simulink model "QAM_16_Transceiver_Nishat"  (R2018a)
settings: Solver=ode45  StartTime=0.0  StopTime=inf  RelTol=1e-3  EnableMultiTasking=on
values from neighbouring files (symbols this model uses):
  FrameTime = 0.000552    [qpsktxrx16.mat]
  qpsktxrx =     [qpsktxrx16.mat]
undefined symbols (not defined in the file or in its folder): dfilt
libraries: simulink x6, dspsigops x6, dspstat3 x6, dspobslib x6, commdigbbndam3 x5, commblkintrlv2 x5, commutil2 x4, commrflib2 x3, dspsrcs4 x3, commfilt2 x3, commblksprivate x2, dspspect3 x2
(part 2 of 3)

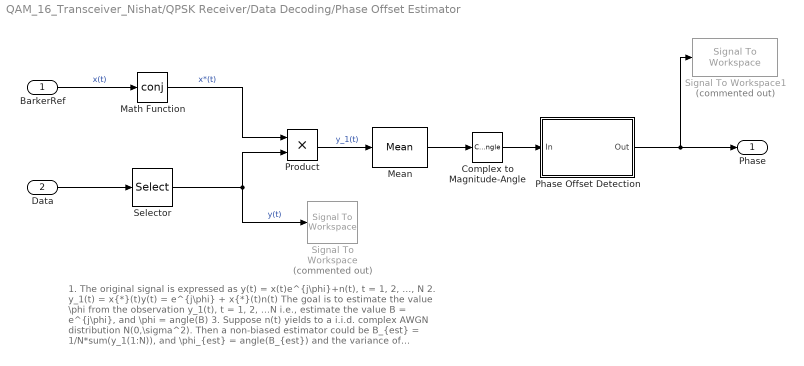
== system QAM_16_Transceiver_Nishat/QPSK Receiver/Data Decoding/Phase Offset Estimator ==
  note: 1. The original signal is expressed as y(t) = x(t)e^{j\phi}+n(t), t = 1, 2, ..., N
      | 2. y_1(t) = x{*}(t)y(t) = e^{j\phi} + x{*}(t)n(t)
      | The goal is to estimate the value \phi from the observation y_1(t), t = 1, 2, ...N
      | i.e., estimate the value B = e^{j\phi}, and \phi = angle(B)
      | 3. Suppose n(t) yields to a i.i.d. complex AWGN distribution N(0,\sigma^2).
      | Then a non-biased estimator could be
      | B_{est} = 1/N*sum(y_1(1:N)), and \phi_{est} = angle(B_{est})
      | and the variance of B_{est} is \sigma^2/N
  BarkerRef : Inport
  Data : Inport  Port=2
  Complex to Magnitude-Angle : ComplexToMagnitudeAngle  Output=Angle
  Math Function : Math  Operator=conj  SaturateOnIntegerOverflow=on
  Mean : dspstat3/Mean  run=off  InputProcessing=Columns as channels (frame based)  reset_popup=None  directionMode=Each column  dimension=1  roiEnable=off  roiType=Rectangles  roiPortion=Entire ROI  roiOutput=Individual statistics for each ROI  roiFlag=off  roundingMode=Floor  overflowMode=off  outputDataTypeStr=Inherit: Same as accumulator  outputMin=[]  outputMax=[]  outputLastDataTypeStr=Inherit: Same as accumulator
  Phase Offset Detection : MATLAB Function  TreatAsAtomicUnit=on
  Product : Product  RndMeth=Zero
  Selector : Selector  IndexOptions=Index vector (dialog)  Indices=[1:26]  OutputSizes=1
  Signal To Workspace : SignalToWorkspace  Commented=on  VariableName=received_Barker
      settings: CopyFcn=dspblkcopystw(gcbh);  Save2DSignal=3-D array (concatenate along third dimension)
  Signal To Workspace1 : SignalToWorkspace  Commented=on  VariableName=Phase_lock_error
      settings: CopyFcn=dspblkcopystw(gcbh);  Save2DSignal=3-D array (concatenate along third dimension)
  Phase : Outport
  wires:
  Data/1 -> Selector/1
  BarkerRef/1 -> Math Function/1  "x(t)"
  Selector/1 -> Product/2, Signal To Workspace/1  "y(t)"
  Math Function/1 -> Product/1  "x*(t)"
  Product/1 -> Mean/1  "y_1(t)"
  Mean/1 -> Complex to Magnitude-Angle/1
  Complex to Magnitude-Angle/1 -> Phase Offset Detection/1(In)
  Phase Offset Detection/1(Out) -> Phase/1, Signal To Workspace1/1

== system QAM_16_Transceiver_Nishat/QPSK Receiver/Fine Frequency Compensation/DDS ==
  note: The digital filter acts as a pure integrator
  In : Inport
  Digital Filter : dspobslib/Digital Filter  TypePopup=IIR (poles & zeros)  IIRFiltStruct=Direct form II transposed  AllPoleFiltStruct=Direct form  FIRFiltStruct=Direct form  CoeffSource=Specify via dialog  NumCoeffs=[0 1]  DenCoeffs=[1 -1]  BiQuadCoeffs=[1 0.3 0.4 1 0.1 0.2]  LatticeCoeffs=[0.2 0.4]  denIgnore=on  FiltPerSampPopup=One filter per frame  IC=0  ICnum=0  ICden=0  roundingMode=Floor  overflowMode=off  ScaleValues=1  scaleValueFracLength=14  stageInFracLength=15  stageOutFracLength=15  FilterSource=Specify via dialog  dfiltObjectName=dfilt.dffir([1 2 1])  InputProcessing=Columns as channels (frame based)
      settings: SourceProductName=DSP System Toolbox  SourceProductBaseCode=DS
  Gain : Gain  Gain=-1*qpsktxrx.PhaseRecoveryGain
  Phase : Outport
  wires:
  Digital Filter/1 -> Gain/1
  In/1 -> Digital Filter/1
  Gain/1 -> Phase/1

== system QAM_16_Transceiver_Nishat/QPSK Receiver/Fine Frequency Compensation/Loop Filter ==
  note: Proportional-plus-Integrator Loop Filter,
      | Infinite DC Response to guarantee convergence
  e : Inport
  Digital Filter : dspobslib/Digital Filter  TypePopup=IIR (poles & zeros)  IIRFiltStruct=Direct form II transposed  AllPoleFiltStruct=Direct form  FIRFiltStruct=Direct form  CoeffSource=Specify via dialog  NumCoeffs=[1 0]  DenCoeffs=[1 -1]  BiQuadCoeffs=[1 0.3 0.4 1 0.1 0.2]  LatticeCoeffs=[0.2 0.4]  denIgnore=on  FiltPerSampPopup=One filter per frame  IC=0  ICnum=0  ICden=0  roundingMode=Floor  overflowMode=off  ScaleValues=1  scaleValueFracLength=14  stageInFracLength=15  stageOutFracLength=15  FilterSource=Specify via dialog  dfiltObjectName=dfilt.dffir([1 2 1])  InputProcessing=Columns as channels (frame based)
      settings: SourceProductName=DSP System Toolbox  SourceProductBaseCode=DS
  K1 : Gain  Gain=K1
  K2 : Gain  Gain=K2
  Sum2 : Sum  SaturateOnIntegerOverflow=on  InputSameDT=on  OutDataTypeStr=Inherit: Same as first input
  v : Outport
  wires:
  K2/1 -> Digital Filter/1
  Digital Filter/1 -> Sum2/2
  Sum2/1 -> v/1
  e/1 -> K2/1, K1/1
  K1/1 -> Sum2/1

== system QAM_16_Transceiver_Nishat/QPSK Receiver/Timing Recovery/Enabled Wire ==
  In : Inport
  Enable : EnablePort
  Out : Outport
  wires:
  In/1 -> Out/1

== system QAM_16_Transceiver_Nishat/QPSK Receiver/Timing Recovery/Modified Buffer ==
  Data : Inport
  Clk : Inport  Port=2
  Frame Conversion : FrameConversion  OutFrame=Sample-based
  Logical Operator : Logic  AllPortsSameDT=off  OutDataTypeStr=boolean
  Modified Buffer : Subsystem
  DataOut : Outport
  DataValid : Outport  Port=2
  wires:
  Data/1 -> Modified Buffer/1(In)
  Modified Buffer/1(DataOut) -> Frame Conversion/1
  Modified Buffer/2(DataValid) -> Logical Operator/1
  Logical Operator/1 -> DataValid/1
  Frame Conversion/1 -> DataOut/1
  Clk/1 -> Modified Buffer/Enable, Logical Operator/2

== system QAM_16_Transceiver_Nishat/QPSK Receiver/Timing Recovery/Timing Recovery PLL ==
  note: Sample-based processing is adopted because
      | 1. Strobe signal is required to generate for EVERY sample for processing and output
      | sampling, delayed strobe signal would affect the accuracy of bit stripping/stuffing
      | 2. The BER performance degrades significantly even with frame size 2 and 4
  note: Baseband implementation of the Symbol Timing Synchronization listed in Chapter 8.4
      | of "Digital Communications- A Discrete-Time Approach" by Michael Rice. See Appendix
      | C.2 of the same book for the details of PLL design.
  note: To determine phase error detector gain K_p, See Equation 8.42 &
      | Figure 8.4.7 of "Digital Communications - A Discrete-Time Approach"
      | by Michael Rice.
  DataIn : Inport
  Integer Delay1 : Delay  DelayLength=1  InputProcessing=Inherited
  Integer Delay2 : Delay  DelayLength=1  InputProcessing=Inherited
  Interpolation Filter : MATLAB Function  TreatAsAtomicUnit=on
  Loop Filter : Subsystem  mask{BnTs=0.01, zeta=1, Kp=qpsktxrx.TimingErrorDetectorGain, K0=qpsktxrx.TimingRecoveryGain, N=qpsktxrx.Upsampling/qpsktxrx.Downsampling}
      mask prompts: BnTs "Loop Bandwidth"; zeta "Loop Damping Factor"; Kp "Phase Detector Gain (Kp)"; K0 "DDS gain (K0)"; N "Number of Samples/symbol (N)"
      mask init:
      | % See C.57 to C.61 in Michael Rice's "Digital Communications 
      | % - A Discrete-Time Approach" for details
      | theta = BnTs/(zeta+0.25/zeta)/N;
      | d = 1 + 2*zeta*theta + theta*theta;
      | K1 = 4*zeta*theta/d;
      | K2 = 4*theta*theta/d;
      | K1 = K1/(Kp*K0);
      | K2 = K2/(Kp*K0);
      mask Display: disp('Loop Filter');
  NCO Control : MATLAB Function
  Normalized Timing Error : Scope
  Timing Error Detector : MATLAB Function  TreatAsAtomicUnit=on
  DataOut : Outport
  ClkOut : Outport  Port=2
  wires:
  DataIn/1 -> Interpolation Filter/1(In)
  NCO Control/2(mu) -> Integer Delay2/1
  Integer Delay1/1 -> ClkOut/1, Timing Error Detector/2(strobe)
  NCO Control/1(Underflow) -> Integer Delay1/1
  Interpolation Filter/1(Out) -> DataOut/1, Timing Error Detector/1(In)
  Loop Filter/1(v) -> NCO Control/1(Delta)
  Timing Error Detector/1(e) -> Loop Filter/1(e)
  Integer Delay2/1 -> Interpolation Filter/2(mu), Normalized Timing Error/1

== system QAM_16_Transceiver_Nishat/Receiver/Coarse Frequency Compensation/Find Frequency Offset ==
  note: This subsystem does the following:
      | 1.  Creates a tone at M*Foffset, where M is the modulation order of the signal
      | 2.  Finds the index of the maximum amplitude across the frequency band
      | 3.  Converts the index to the frequency offset according to
      | Foffset = IndexofMaxAmplitude * FrameSize / (FFTLength * M * FrameSampleTime)
  In : Inport
  Alphabet size : Constant  Value=4  OutDataTypeStr=Inherit: Inherit via back propagation
  Complex Power : commblksprivate/Complex Power
      settings: SourceProductName=Communications System Toolbox  SourceProductBaseCode=CM
  Find Frequency Offset : MATLAB Function  TreatAsAtomicUnit=on
  Periodogram : dspspect3/Periodogram  measurement=Power spectral density  wintype=Hamming  Rs=50  beta=5  winsamp=Symmetric  FFTImplementation=Auto  inheritFFT=off  fftsize=2048  navg=2  inheritTs=on  Ts=1
      settings: SourceProductName=DSP System Toolbox  SourceProductBaseCode=DS
  Probe : Probe  ProbeComplexSignal=off
  Signal To Workspace : SignalToWorkspace  Commented=on  VariableName=width
      settings: CopyFcn=dspblkcopystw(gcbh);  Save2DSignal=3-D array (concatenate along third dimension)
  Freq Offset : Outport
  wires:
  Periodogram/1 -> Find Frequency Offset/3(FFTSig)
  Alphabet size/1 -> Complex Power/2
  In/1 -> Complex Power/1
  Probe/1 -> Find Frequency Offset/1(N)
  Probe/2 -> Find Frequency Offset/2(Tf)
  Find Frequency Offset/1(FreqOffset) -> Signal To Workspace/1, Freq Offset/1
  Complex Power/1 -> Probe/1, Periodogram/1

== system QAM_16_Transceiver_Nishat/Receiver/Data Decoding/Barker Code Symbol Generation  ==
  note: Regenerate a QPSK-modulated unipolar Barker code sequence
      | to be compared with the received data
  Constant Barker Code : Constant  Value=|  VectorParams1D=off  OutDataTypeStr=double
      | [+1 +1 +1 +1 +1 -1 -1 +1 +1 -1 +1 -1 +1
      | ].' > 0
  Matrix Concatenate : Concatenate  Mode=Multidimensional array
  Rectangular QAM Modulator Baseband : commdigbbndam3/Rectangular QAM Modulator Baseband  M=16  InType=Bit  Enc=Gray  Mapping=[0:15]  PowType=Min. distance between symbols  MinDist=2  AvgPow=1  PeakPow=1  Ph=0  outDtype=double  outWordLen=16  outUDDataType=sfix(16)  outFracLenMode=Best precision  outFracLen=15  outDataTypeStr=double  outLastDataTypeStr=double
  Repeat : dspsigops/Repeat  N=4  InputProcessing=Columns as channels (frame based)  RateOptions=Enforce single-rate processing  ic=0  mode=Unused parameter value
      settings: SourceProductName=DSP System Toolbox
  Out : Outport
  wires:
  Constant Barker Code/1 -> Repeat/1
  Repeat/1 -> Rectangular QAM Modulator Baseband/1
  Rectangular QAM Modulator Baseband/1 -> Matrix Concatenate/2, Matrix Concatenate/1
  Matrix Concatenate/1 -> Out/1

== system QAM_16_Transceiver_Nishat/Receiver/Data Decoding/Bit Generation ==
  note: Each data frame contains 26 bits header (For Sync Purpose) and 174 bits data bits,
      | first 105 bits contain "Hello world ###" message. Scrambler is there to improve data
      | transition density and frequency offset estimation.
  Barker Code SS : Subsystem
      mask Display: disp('Unipolar\nBarker Code')
  Frame Conversion : FrameConversion  OutFrame=Sample-based
  Matrix Concatenate : Concatenate  NumInputs=3  Mode=Multidimensional array
  Random Interleaver : commblkintrlv2/Random Interleaver  N=qpsktxrx.DataLength  seed=12345
      settings: SourceProductName=Communications System Toolbox  SourceProductBaseCode=CM
  Repeat : dspsigops/Repeat  N=4  InputProcessing=Columns as channels (frame based)  RateOptions=Enforce single-rate processing  ic=0  mode=Unused parameter value
      settings: SourceProductName=DSP System Toolbox
  Signal From Workspace : dspsrcs4/Signal From Workspace  X=qpsktxrx.sBit2  Ts=-1  nsamps=qpsktxrx.DataLength  OutputAfterFinalValue=Cyclic repetition  ignoreOrWarnInputAndFrameLengths=off  OutputFrames=on
  Out : Outport
  wires:
  Frame Conversion/1 -> Random Interleaver/1
  Repeat/1 -> Matrix Concatenate/2, Matrix Concatenate/1
  Signal From Workspace/1 -> Frame Conversion/1
  Matrix Concatenate/1 -> Out/1
  Barker Code SS/1(Out) -> Repeat/1
  Random Interleaver/1 -> Matrix Concatenate/3

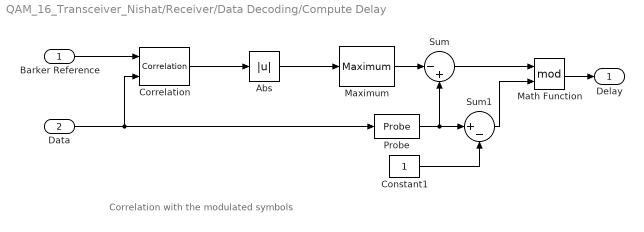
== system QAM_16_Transceiver_Nishat/Receiver/Data Decoding/Compute Delay ==
  note: Correlation with the modulated symbols
  Barker Reference : Inport
  Data : Inport  Port=2
  Abs : Abs
  Constant1 : Constant  VectorParams1D=off  OutDataTypeStr=Inherit: Inherit via back propagation  FramePeriod=2
  Correlation : dspstat3/Correlation  domain=Time  roundingMode=Floor  overflowMode=off  accumDataTypeStr=Inherit: Same as product output  accumLastDataTypeStr=Inherit: Same as product output  outputDataTypeStr=Inherit: Same as accumulator  outputMin=[]  outputMax=[]  outputLastDataTypeStr=Inherit: Same as accumulator
      settings: SourceProductName=DSP System Toolbox  SourceProductBaseCode=DS
  Math Function : Math  Operator=mod  SaturateOnIntegerOverflow=on
  Maximum : dspstat3/Maximum  operation=maximum  fcn=Index  indexBase=One  operateOver=Each column  Dimension=1  InputProcessing=Columns as channels (frame based)  reset=None  roiEnable=off  roiType=Rectangles  roiPortion=Entire ROI  roiOutput=Individual statistics for each ROI  roiFlag=off  roundingMode=Floor  overflowMode=off  accumDataTypeStr=Inherit: Same as product output  accumLastDataTypeStr=Inherit: Same as product output
  Probe : Probe  ProbeSampleTime=off  ProbeComplexSignal=off
  Sum : Sum  Inputs=|-+  SaturateOnIntegerOverflow=on  InputSameDT=on  OutDataTypeStr=Inherit: Same as first input
  Sum1 : Sum  Inputs=|+-  SaturateOnIntegerOverflow=on  InputSameDT=on  OutDataTypeStr=Inherit: Same as first input
  Delay : Outport
  wires:
  Abs/1 -> Maximum/1
  Constant1/1 -> Sum1/2
  Sum1/1 -> Math Function/2
  Math Function/1 -> Delay/1
  Sum/1 -> Math Function/1
  Probe/1 -> Sum1/1, Sum/2
  Correlation/1 -> Abs/1
  Maximum/1 -> Sum/1
  Barker Reference/1 -> Correlation/1
  Data/1 -> Correlation/2, Probe/1

== system QAM_16_Transceiver_Nishat/Receiver/Data Decoding/Descrambling ==
  In : Inport
  Random Deinterleaver : commblkintrlv2/Random Deinterleaver  N=qpsktxrx.DataLength  seed=12345
      settings: SourceProductName=Communications System Toolbox  SourceProductBaseCode=CM
  Selector : Selector  IndexOptions=Index vector (dialog)  Indices=[qpsktxrx.BarkerLength*log2(qpsktxrx.M)+1:qpsktxrx.FrameSize*log2(qpsktxrx.M)]  OutputSizes=1
  Signal To Workspace : SignalToWorkspace  Commented=on  VariableName=after_deinterleaver
      settings: CopyFcn=dspblkcopystw(gcbh);
  Signal To Workspace1 : SignalToWorkspace  Commented=on  VariableName=before_deinterleaver
      settings: CopyFcn=dspblkcopystw(gcbh);
  Signal To Workspace2 : SignalToWorkspace  Commented=on  VariableName=received_complete
      settings: CopyFcn=dspblkcopystw(gcbh);
  Out : Outport
  wires:
  Selector/1 -> Random Deinterleaver/1, Signal To Workspace1/1
  In/1 -> Signal To Workspace2/1, Selector/1
  Random Deinterleaver/1 -> Out/1, Signal To Workspace/1

== system QAM_16_Transceiver_Nishat/Receiver/Data Decoding/Phase Ambiguity Correction & Demodulation ==
  note: Phase Ambiguity Resolution
      | and Demodulation
  Phase : Inport
  Data : Inport  Port=2
  Complex Phase Shift : commutil2/Complex Phase Shift
      settings: SourceProductName=Communications System Toolbox  SourceProductBaseCode=CM
  Corrected Symbols : ConstellationDiagram  Tag=ScatterPlot
  Gain : Gain  Gain=-1  OutDataTypeStr=Inherit: Same as input
  Probe2 : Probe  ProbeSampleTime=off  ProbeComplexSignal=off
  Rectangular QAM Demodulator Baseband : commdigbbndam3/Rectangular QAM Demodulator Baseband  M=16  OutType=Bit  DecType=Hard decision  VarSource=Dialog  Variance=1  Dec=Gray  Mapping=[0:15]  PowType=Min. distance between symbols  MinDist=2  AvgPow=1  PeakPow=1  Ph=0  outDtype1=Inherit via internal rule  outDtype2=Inherit via internal rule  derotateFactorWordLen=16  derotateFactorDataTypeStr=Inherit: Same word length as input  derotateFactorLastDataTypeStr=Inherit: Same word length as input  denormFactorWordLen=16  denormFactorDataTypeStr=Inherit: Same word length as input  denormFactorLastDataTypeStr=Inherit: Same word length as input  prodOutWordLen=32  prodOutOverflowMode=Wrap  prodOutRoundingMode=Floor  prodOutOvFlMode=off  prodOutOvFlModeLastStrValue=off  sumWordLen=32
  Signal To Workspace2 : SignalToWorkspace  Commented=on  VariableName=after_phase_ambiguity
      settings: CopyFcn=dspblkcopystw(gcbh);
  Out : Outport
  wires:
  Phase/1 -> Gain/1
  Complex Phase Shift/1 -> Signal To Workspace2/1, Probe2/1, Corrected Symbols/1, Rectangular QAM Demodulator Baseband/1
  Rectangular QAM Demodulator Baseband/1 -> Out/1
  Gain/1 -> Complex Phase Shift/2
  Data/1 -> Complex Phase Shift/1

== system QAM_16_Transceiver_Nishat/Receiver/Data Decoding/Phase Offset Estimator ==
  note: 1. The original signal is expressed as y(t) = x(t)e^{j\phi}+n(t), t = 1, 2, ..., N
      | 2. y_1(t) = x{*}(t)y(t) = e^{j\phi} + x{*}(t)n(t)
      | The goal is to estimate the value \phi from the observation y_1(t), t = 1, 2, ...N
      | i.e., estimate the value B = e^{j\phi}, and \phi = angle(B)
      | 3. Suppose n(t) yields to a i.i.d. complex AWGN distribution N(0,\sigma^2).
      | Then a non-biased estimator could be
      | B_{est} = 1/N*sum(y_1(1:N)), and \phi_{est} = angle(B_{est})
      | and the variance of B_{est} is \sigma^2/N
  BarkerRef : Inport
  Data : Inport  Port=2
  Complex to Magnitude-Angle : ComplexToMagnitudeAngle  Output=Angle
  Math Function : Math  Operator=conj  SaturateOnIntegerOverflow=on
  Mean : dspstat3/Mean  run=off  InputProcessing=Columns as channels (frame based)  reset_popup=None  directionMode=Each column  dimension=1  roiEnable=off  roiType=Rectangles  roiPortion=Entire ROI  roiOutput=Individual statistics for each ROI  roiFlag=off  roundingMode=Floor  overflowMode=off  outputDataTypeStr=Inherit: Same as accumulator  outputMin=[]  outputMax=[]  outputLastDataTypeStr=Inherit: Same as accumulator
  Phase Offset Detection : MATLAB Function  TreatAsAtomicUnit=on
  Product : Product  RndMeth=Zero
  Selector : Selector  IndexOptions=Index vector (dialog)  Indices=[1:26]  OutputSizes=1
  Signal To Workspace : SignalToWorkspace  Commented=on  VariableName=received_Barker
      settings: CopyFcn=dspblkcopystw(gcbh);  Save2DSignal=3-D array (concatenate along third dimension)
  Signal To Workspace1 : SignalToWorkspace  Commented=on  VariableName=Phase_lock_error
      settings: CopyFcn=dspblkcopystw(gcbh);  Save2DSignal=3-D array (concatenate along third dimension)
  Phase : Outport
  wires:
  Data/1 -> Selector/1
  BarkerRef/1 -> Math Function/1  "x(t)"
  Selector/1 -> Product/2, Signal To Workspace/1  "y(t)"
  Math Function/1 -> Product/1  "x*(t)"
  Product/1 -> Mean/1  "y_1(t)"
  Mean/1 -> Complex to Magnitude-Angle/1
  Complex to Magnitude-Angle/1 -> Phase Offset Detection/1(In)
  Phase Offset Detection/1(Out) -> Phase/1, Signal To Workspace1/1

== system QAM_16_Transceiver_Nishat/Receiver/Fine Frequency Compensation/DDS ==
  note: The digital filter acts as a pure integrator
  In : Inport
  Digital Filter : dspobslib/Digital Filter  TypePopup=IIR (poles & zeros)  IIRFiltStruct=Direct form II transposed  AllPoleFiltStruct=Direct form  FIRFiltStruct=Direct form  CoeffSource=Specify via dialog  NumCoeffs=[0 1]  DenCoeffs=[1 -1]  BiQuadCoeffs=[1 0.3 0.4 1 0.1 0.2]  LatticeCoeffs=[0.2 0.4]  denIgnore=on  FiltPerSampPopup=One filter per frame  IC=0  ICnum=0  ICden=0  roundingMode=Floor  overflowMode=off  ScaleValues=1  scaleValueFracLength=14  stageInFracLength=15  stageOutFracLength=15  FilterSource=Specify via dialog  dfiltObjectName=dfilt.dffir([1 2 1])  InputProcessing=Columns as channels (frame based)
      settings: SourceProductName=DSP System Toolbox  SourceProductBaseCode=DS
  Gain : Gain  Gain=-1*qpsktxrx.PhaseRecoveryGain
  Phase : Outport
  wires:
  Digital Filter/1 -> Gain/1
  In/1 -> Digital Filter/1
  Gain/1 -> Phase/1

== system QAM_16_Transceiver_Nishat/Receiver/Fine Frequency Compensation/Loop Filter ==
  note: Proportional-plus-Integrator Loop Filter,
      | Infinite DC Response to guarantee convergence
  e : Inport
  Digital Filter : dspobslib/Digital Filter  TypePopup=IIR (poles & zeros)  IIRFiltStruct=Direct form II transposed  AllPoleFiltStruct=Direct form  FIRFiltStruct=Direct form  CoeffSource=Specify via dialog  NumCoeffs=[1 0]  DenCoeffs=[1 -1]  BiQuadCoeffs=[1 0.3 0.4 1 0.1 0.2]  LatticeCoeffs=[0.2 0.4]  denIgnore=on  FiltPerSampPopup=One filter per frame  IC=0  ICnum=0  ICden=0  roundingMode=Floor  overflowMode=off  ScaleValues=1  scaleValueFracLength=14  stageInFracLength=15  stageOutFracLength=15  FilterSource=Specify via dialog  dfiltObjectName=dfilt.dffir([1 2 1])  InputProcessing=Columns as channels (frame based)
      settings: SourceProductName=DSP System Toolbox  SourceProductBaseCode=DS
  K1 : Gain  Gain=K1
  K2 : Gain  Gain=K2
  Sum2 : Sum  SaturateOnIntegerOverflow=on  InputSameDT=on  OutDataTypeStr=Inherit: Same as first input
  v : Outport
  wires:
  K2/1 -> Digital Filter/1
  Digital Filter/1 -> Sum2/2
  Sum2/1 -> v/1
  e/1 -> K2/1, K1/1
  K1/1 -> Sum2/1

== system QAM_16_Transceiver_Nishat/Receiver/Timing Recovery/Enabled Wire ==
  In : Inport
  Enable : EnablePort
  Out : Outport
  wires:
  In/1 -> Out/1

== system QAM_16_Transceiver_Nishat/Receiver/Timing Recovery/Modified Buffer ==
  Data : Inport
  Clk : Inport  Port=2
  Frame Conversion : FrameConversion  OutFrame=Sample-based
  Logical Operator : Logic  AllPortsSameDT=off  OutDataTypeStr=boolean
  Modified Buffer : Subsystem
  DataOut : Outport
  DataValid : Outport  Port=2
  wires:
  Data/1 -> Modified Buffer/1(In)
  Modified Buffer/1(DataOut) -> Frame Conversion/1
  Modified Buffer/2(DataValid) -> Logical Operator/1
  Logical Operator/1 -> DataValid/1
  Frame Conversion/1 -> DataOut/1
  Clk/1 -> Modified Buffer/Enable, Logical Operator/2

== system QAM_16_Transceiver_Nishat/Receiver/Timing Recovery/Timing Recovery PLL ==
  note: Sample-based processing is adopted because
      | 1. Strobe signal is required to generate for EVERY sample for processing and output
      | sampling, delayed strobe signal would affect the accuracy of bit stripping/stuffing
      | 2. The BER performance degrades significantly even with frame size 2 and 4
  note: Baseband implementation of the Symbol Timing Synchronization listed in Chapter 8.4
      | of "Digital Communications- A Discrete-Time Approach" by Michael Rice. See Appendix
      | C.2 of the same book for the details of PLL design.
  note: To determine phase error detector gain K_p, See Equation 8.42 &
      | Figure 8.4.7 of "Digital Communications - A Discrete-Time Approach"
      | by Michael Rice.
  DataIn : Inport
  Integer Delay1 : Delay  DelayLength=1  InputProcessing=Inherited
  Integer Delay2 : Delay  DelayLength=1  InputProcessing=Inherited
  Interpolation Filter : MATLAB Function  TreatAsAtomicUnit=on
  Loop Filter : Subsystem  mask{BnTs=0.01, zeta=1, Kp=qpsktxrx.TimingErrorDetectorGain, K0=qpsktxrx.TimingRecoveryGain, N=qpsktxrx.Upsampling/qpsktxrx.Downsampling}
      mask prompts: BnTs "Loop Bandwidth"; zeta "Loop Damping Factor"; Kp "Phase Detector Gain (Kp)"; K0 "DDS gain (K0)"; N "Number of Samples/symbol (N)"
      mask init: same as QAM_16_Transceiver_Nishat/QPSK Receiver/Timing Recovery/Timing Recovery PLL/Loop Filter
      mask Display: disp('Loop Filter');
  NCO Control : MATLAB Function
  Normalized Timing Error : Scope
  Timing Error Detector : MATLAB Function  TreatAsAtomicUnit=on
  DataOut : Outport
  ClkOut : Outport  Port=2
  wires:
  DataIn/1 -> Interpolation Filter/1(In)
  NCO Control/2(mu) -> Integer Delay2/1
  Integer Delay1/1 -> ClkOut/1, Timing Error Detector/2(strobe)
  NCO Control/1(Underflow) -> Integer Delay1/1
  Interpolation Filter/1(Out) -> DataOut/1, Timing Error Detector/1(In)
  Loop Filter/1(v) -> NCO Control/1(Delta)
  Timing Error Detector/1(e) -> Loop Filter/1(e)
  Integer Delay2/1 -> Interpolation Filter/2(mu), Normalized Timing Error/1

== system QAM_16_Transceiver_Nishat/Transmitter/Bit Generation/Barker Code SS ==
  Constant Barker Code : Constant  Value=|  VectorParams1D=off  OutDataTypeStr=double
      | [+1 +1 +1 +1 +1 -1 -1 +1 +1 -1 +1 -1 +1
      | ].' > 0  % Bipolar to Unipolar Conversion
  Out : Outport
  wires:
  Constant Barker Code/1 -> Out/1

== system QAM_16_Transceiver_Nishat/QPSK Receiver/Data Decoding/Bit Generation/Barker Code SS ==
  Constant Barker Code : Constant  Value=|  VectorParams1D=off  OutDataTypeStr=double
      | [+1 +1 +1 +1 +1 -1 -1 +1 +1 -1 +1 -1 +1
      | ].' > 0  % Bipolar to Unipolar Conversion
  Out : Outport
  wires:
  Constant Barker Code/1 -> Out/1

== system QAM_16_Transceiver_Nishat/QPSK Receiver/Timing Recovery/Modified Buffer/Modified Buffer ==
  In : Inport
  Enable : EnablePort
  Compare To Constant : simulink/Logic and Bit Operations/Compare To Constant  relop===  const=(bufSize-1)  OutDataTypeStr=boolean  ZeroCross=off
  Counter Limited : simulink/Sources/Counter Limited  uplimit=(bufSize-1)  tsamp=-1
  Delay Line : dspbuff3/Delay Line  siz=bufSize  ic=0  directfeed=on  enable_output=on  hold_output=off  OutputFrames=on
      settings: SourceProductName=DSP System Toolbox  SourceProductBaseCode=DS
  DataOut : Outport
  DataValid : Outport  Port=2
  wires:
  Compare To Constant/1 -> Delay Line/2, DataValid/1
  Delay Line/1 -> DataOut/1
  In/1 -> Delay Line/1
  Counter Limited/1 -> Compare To Constant/1

== system QAM_16_Transceiver_Nishat/QPSK Receiver/Timing Recovery/Timing Recovery PLL/Loop Filter ==
  note: Proportional-Plus-Integrator Loop Filter,
      | Infinite DC Response to guarantee convergence
  e : Inport
  Digital Filter : dspobslib/Digital Filter  TypePopup=IIR (poles & zeros)  IIRFiltStruct=Direct form II transposed  AllPoleFiltStruct=Direct form  FIRFiltStruct=Direct form  CoeffSource=Specify via dialog  NumCoeffs=[1 0]  DenCoeffs=[1 -1]  BiQuadCoeffs=[1 0.3 0.4 1 0.1 0.2]  LatticeCoeffs=[0.2 0.4]  denIgnore=on  FiltPerSampPopup=One filter per frame  IC=0  ICnum=0  ICden=0  roundingMode=Floor  overflowMode=off  ScaleValues=1  scaleValueFracLength=14  stageInFracLength=15  stageOutFracLength=15  FilterSource=Specify via dialog  dfiltObjectName=dfilt.dffir([1 2 1])  InputProcessing=Columns as channels (frame based)
      settings: SourceProductName=DSP System Toolbox  SourceProductBaseCode=DS
  K1 : Gain  Gain=K1
  K2 : Gain  Gain=K2
  Sum2 : Sum  SaturateOnIntegerOverflow=on  InputSameDT=on  OutDataTypeStr=Inherit: Same as first input
  v : Outport
  wires:
  K2/1 -> Digital Filter/1
  Digital Filter/1 -> Sum2/2
  Sum2/1 -> v/1
  e/1 -> K2/1, K1/1
  K1/1 -> Sum2/1

== system QAM_16_Transceiver_Nishat/Receiver/Data Decoding/Bit Generation/Barker Code SS ==
  Constant Barker Code : Constant  Value=|  VectorParams1D=off  OutDataTypeStr=double
      | [+1 +1 +1 +1 +1 -1 -1 +1 +1 -1 +1 -1 +1
      | ].' > 0  % Bipolar to Unipolar Conversion
  Out : Outport
  wires:
  Constant Barker Code/1 -> Out/1

== system QAM_16_Transceiver_Nishat/Receiver/Timing Recovery/Modified Buffer/Modified Buffer ==
  In : Inport
  Enable : EnablePort
  Compare To Constant : simulink/Logic and Bit Operations/Compare To Constant  relop===  const=(bufSize-1)  OutDataTypeStr=boolean  ZeroCross=off
  Counter Limited : simulink/Sources/Counter Limited  uplimit=(bufSize-1)  tsamp=-1
  Delay Line : dspbuff3/Delay Line  siz=bufSize  ic=0  directfeed=on  enable_output=on  hold_output=off  OutputFrames=on
      settings: SourceProductName=DSP System Toolbox  SourceProductBaseCode=DS
  DataOut : Outport
  DataValid : Outport  Port=2
  wires:
  Compare To Constant/1 -> Delay Line/2, DataValid/1
  Delay Line/1 -> DataOut/1
  In/1 -> Delay Line/1
  Counter Limited/1 -> Compare To Constant/1

== system QAM_16_Transceiver_Nishat/Receiver/Timing Recovery/Timing Recovery PLL/Loop Filter ==
  note: Proportional-Plus-Integrator Loop Filter,
      | Infinite DC Response to guarantee convergence
  e : Inport
  Digital Filter : dspobslib/Digital Filter  TypePopup=IIR (poles & zeros)  IIRFiltStruct=Direct form II transposed  AllPoleFiltStruct=Direct form  FIRFiltStruct=Direct form  CoeffSource=Specify via dialog  NumCoeffs=[1 0]  DenCoeffs=[1 -1]  BiQuadCoeffs=[1 0.3 0.4 1 0.1 0.2]  LatticeCoeffs=[0.2 0.4]  denIgnore=on  FiltPerSampPopup=One filter per frame  IC=0  ICnum=0  ICden=0  roundingMode=Floor  overflowMode=off  ScaleValues=1  scaleValueFracLength=14  stageInFracLength=15  stageOutFracLength=15  FilterSource=Specify via dialog  dfiltObjectName=dfilt.dffir([1 2 1])  InputProcessing=Columns as channels (frame based)
      settings: SourceProductName=DSP System Toolbox  SourceProductBaseCode=DS
  K1 : Gain  Gain=K1
  K2 : Gain  Gain=K2
  Sum2 : Sum  SaturateOnIntegerOverflow=on  InputSameDT=on  OutDataTypeStr=Inherit: Same as first input
  v : Outport
  wires:
  K2/1 -> Digital Filter/1
  Digital Filter/1 -> Sum2/2
  Sum2/1 -> v/1
  e/1 -> K2/1, K1/1
  K1/1 -> Sum2/1

== matlab function QAM_16_Transceiver_Nishat/QPSK Receiver/Auto correlation ==
  data: frame input; frame_length input; output output; auto_corr_length input; Status_value output; Status_position output; MaximumValue output; SecondMaximumValue output; Index output; MaximumIndex output; correction_factor output
 function [output , Status_value , Status_position , MaximumValue , SecondMaximumValue , Index , MaximumIndex , correction_factor]  = auto_corr(frame , frame_length , auto_corr_length)

% This block is data aided preamble based AGC. This can work with any M-QAM
% constellation.

output = complex(zeros(552,1));
frame = frame.';

num_auto_corr = frame_length - 2*auto_corr_length + 1;
assert(num_auto_corr < 2048);
auto_corr_array = complex(zeros(1,num_auto_corr));
auto_corr_array_mag = zeros(1,num_auto_corr);

temp = complex(0);

for i = 1:num_auto_corr
    
    if (i==1)
    
        auto_corr_array(i) = temp + frame(i:auto_corr_length)*((frame(auto_corr_length + i : 2*auto_corr_length)))';    % " ' " used to avoid using sum --> multiplicatin of row and column array
        auto_corr_array_mag(i) = abs(auto_corr_array(i));
        
        temp = auto_corr_array(i) - ( frame(i) * conj(frame(auto_corr_length+i)) );
    
    elseif (i > 1 )
        
        auto_corr_array(i) = temp + (frame(i-1 + auto_corr_length) * conj(frame(i-1 + auto_corr_length*2)) );    % i-1 bcoz when i = 2 then 14 sample should be * with 27 sample not 15 with 28 
        auto_corr_array_mag(i) = abs(auto_corr_array(i));
        
        temp = auto_corr_array(i) - (frame(i) * conj(frame(auto_corr_length + i)) );
    
    else
        disp('NARGIN ERROR ;)');
    end

end

%% confirmation and estimation process
Status_value = 1;
Status_position = 1;
temp_auto_mag = auto_corr_array_mag;

[MaximumValue, MaximumIndex] = max(temp_auto_mag);
MinThresholdIndex = MaximumIndex;
MaxThresholdIndex = MaximumIndex;

Threshold = 0.8*MaximumValue;

LengthData = num_auto_corr;

temp_auto_mag(MaximumIndex) = -100;

for Index = 1:LengthData
    
    if MinThresholdIndex ~= MaximumIndex && MaxThresholdIndex ~= MaximumIndex
        break;
    end
    
    if MaximumIndex-Index >= 1 && MinThresholdIndex == MaximumIndex && temp_auto_mag(MaximumIndex-Index) < Threshold
        MinThresholdIndex = MaximumIndex-Index+1;
    else
        if MinThresholdIndex == MaximumIndex  && MaximumIndex-Index >= 1
        temp_auto_mag(MaximumIndex-Index) = -100;
        end
    end
    
    if MaximumIndex+Index <= LengthData && MaxThresholdIndex == MaximumIndex && temp_auto_mag(MaximumIndex+Index) < Threshold
        MaxThresholdIndex = MaximumIndex+Index-1;
    else
        if MaxThresholdIndex == MaximumIndex && MaximumIndex+Index <= LengthData
        temp_auto_mag(MaximumIndex+Index) = -100;
        end
    end
    
end



[SecondMaximumValue, Index] = max(temp_auto_mag);

if temp_auto_mag(Index) < 0.85*MaximumValue || temp_auto_mag(Index) > 1.15*MaximumValue
    fprintf('ERROR: Large Difference in Preamble Cross Corelation Values\n');
    Status_value = 0;
end

if abs(Index-MaximumIndex) < (frame_length/2 - 16) || abs(Index-MaximumIndex) > (frame_length/2 + 16)
    fprintf('ERROR: Preamlbe Positions Mismatach\n');
    Status_position = 0;
end
% the value of 212 is chosen because it is the autocorrelation for reference constellation
correction_factor = sqrt(complex(212/(SecondMaximumValue + MaximumValue))); %sqrt because a factor alpha in mag transslated to alpha^2 in auto
correction_factor = real(correction_factor); 

output = (frame.')*correction_factor;%/correction_factor;

return;

end

== matlab function QAM_16_Transceiver_Nishat/Channel model/MATLAB Function ==
  data: u input; y output
function y = ChannelMag(u)
% Rangom channel magnitude for each iteration
scale = 1+.1*rand;

y = u*scale;

== matlab function QAM_16_Transceiver_Nishat/Receiver/Auto correlation ==
  data: frame input; frame_length input; output output; auto_corr_length input; Status_value output; Status_position output; MaximumValue output; SecondMaximumValue output; Index output; MaximumIndex output; correction_factor output
 function [output , Status_value , Status_position , MaximumValue , SecondMaximumValue , Index , MaximumIndex , correction_factor]  = auto_corr(frame , frame_length , auto_corr_length)

% This block is data aided preamble based AGC. This can work with any M-QAM
% constellation.

output = complex(zeros(552,1));
frame = frame.';

num_auto_corr = frame_length - 2*auto_corr_length + 1;
assert(num_auto_corr < 2048);
auto_corr_array = complex(zeros(1,num_auto_corr));
auto_corr_array_mag = zeros(1,num_auto_corr);

temp = complex(0);

for i = 1:num_auto_corr
    
    if (i==1)
    
        auto_corr_array(i) = temp + frame(i:auto_corr_length)*((frame(auto_corr_length + i : 2*auto_corr_length)))';    % " ' " used to avoid using sum --> multiplicatin of row and column array
        auto_corr_array_mag(i) = abs(auto_corr_array(i));
        
        temp = auto_corr_array(i) - ( frame(i) * conj(frame(auto_corr_length+i)) );
    
    elseif (i > 1 )
        
        auto_corr_array(i) = temp + (frame(i-1 + auto_corr_length) * conj(frame(i-1 + auto_corr_length*2)) );    % i-1 bcoz when i = 2 then 14 sample should be * with 27 sample not 15 with 28 
        auto_corr_array_mag(i) = abs(auto_corr_array(i));
        
        temp = auto_corr_array(i) - (frame(i) * conj(frame(auto_corr_length + i)) );
    
    else
        disp('NARGIN ERROR ;)');
    end

end

%% confirmation and estimation process
Status_value = 1;
Status_position = 1;
temp_auto_mag = auto_corr_array_mag;

[MaximumValue, MaximumIndex] = max(temp_auto_mag);
MinThresholdIndex = MaximumIndex;
MaxThresholdIndex = MaximumIndex;

Threshold = 0.8*MaximumValue;

LengthData = num_auto_corr;

temp_auto_mag(MaximumIndex) = -100;

for Index = 1:LengthData
    
    if MinThresholdIndex ~= MaximumIndex && MaxThresholdIndex ~= MaximumIndex
        break;
    end
    
    if MaximumIndex-Index >= 1 && MinThresholdIndex == MaximumIndex && temp_auto_mag(MaximumIndex-Index) < Threshold
        MinThresholdIndex = MaximumIndex-Index+1;
    else
        if MinThresholdIndex == MaximumIndex  && MaximumIndex-Index >= 1
        temp_auto_mag(MaximumIndex-Index) = -100;
        end
    end
    
    if MaximumIndex+Index <= LengthData && MaxThresholdIndex == MaximumIndex && temp_auto_mag(MaximumIndex+Index) < Threshold
        MaxThresholdIndex = MaximumIndex+Index-1;
    else
        if MaxThresholdIndex == MaximumIndex && MaximumIndex+Index <= LengthData
        temp_auto_mag(MaximumIndex+Index) = -100;
        end
    end
    
end



[SecondMaximumValue, Index] = max(temp_auto_mag);

if temp_auto_mag(Index) < 0.85*MaximumValue || temp_auto_mag(Index) > 1.15*MaximumValue
    fprintf('ERROR: Large Difference in Preamble Cross Corelation Values\n');
    Status_value = 0;
end

if abs(Index-MaximumIndex) < (frame_length/2 - 16) || abs(Index-MaximumIndex) > (frame_length/2 + 16)
    fprintf('ERROR: Preamlbe Positions Mismatach\n');
    Status_position = 0;
end
% the value of 212 is chosen because it is the autocorrelation for reference constellation
correction_factor = sqrt(complex(212/(SecondMaximumValue + MaximumValue))); %sqrt because a factor alpha in mag transslated to alpha^2 in auto
correction_factor = real(correction_factor); 

output = (frame.')*correction_factor;%/correction_factor;

return;

end

== matlab function QAM_16_Transceiver_Nishat/Receiver/Timing Recovery/Calculate Number of Valid Samples ==
  data: Clk input; numValid output
function numValid = numValidCalc(Clk)
% Calculate the number of valid outputs in the current received frame. The
% typical value is 100 valid outputs in a 200-element frame. However, in
% bit stuffing case we have 101 valid outputs, and in bit stripping case we 
% have 99 valid outputs.
%
% Input:
%   Clk - Strobe signal
% Output:
%   NumValid - Number of valid outputs in the current received frame 
%#codegen
numValid = sum(Clk~=0);

== matlab function QAM_16_Transceiver_Nishat/QPSK Receiver/Coarse Frequency Compensation/Find Frequency Offset/Find Frequency Offset ==
  data: N input; FreqOffset output; Tf input; FFTSig input; qpsktxrx parameter
function FreqOffset  = findfreqoffset(N, Tf, FFTSig, qpsktxrx)
% Find frequency offset
% Input:
%   N - Frame size
%   Tf - Two-element vector:  [Frame time, Offset time]
%   FFTSig - Result of FFT
%   M - Modulation alphabet size
% Output:
%   FreqOffset - Estimated frequency offset
%#codegen

M = qpsktxrx.M; 
FFTSize = length(FFTSig);
FFTSig = fftshift(FFTSig);
[~, maxIdx] = max(FFTSig); % Find index of max magnitude
OffsetIdx = maxIdx-1-FFTSize/2; % Convert to index symmetric with 0
Ts = Tf(1)/N; % Sample time
delta_f = 1/Ts/FFTSize; % Frequency resolution of FFT 
FreqOffset = OffsetIdx*delta_f/4;% Map offset index back to frequency

== matlab function QAM_16_Transceiver_Nishat/QPSK Receiver/Data Decoding/Align Data ==
  data: Delay input; RxData input; Data output
function Data  = aligndata(Delay, RxData)
% Extract data from the buffered RxData, using the delay to find the frame 


Data = RxData(Delay+1:Delay+length(RxData)/2);

== matlab function QAM_16_Transceiver_Nishat/Receiver/Coarse Frequency Compensation/Find Frequency Offset/Find Frequency Offset ==
  data: N input; FreqOffset output; Tf input; FFTSig input; qpsktxrx parameter
function FreqOffset  = findfreqoffset(N, Tf, FFTSig, qpsktxrx)
% Find frequency offset
% Input:
%   N - Frame size
%   Tf - Two-element vector:  [Frame time, Offset time]
%   FFTSig - Result of FFT
%   M - Modulation alphabet size
% Output:
%   FreqOffset - Estimated frequency offset
%#codegen

M = qpsktxrx.M; 
FFTSize = length(FFTSig);
FFTSig = fftshift(FFTSig);
[~, maxIdx] = max(FFTSig); % Find index of max magnitude
OffsetIdx = maxIdx-1-FFTSize/2; % Convert to index symmetric with 0
Ts = Tf(1)/N; % Sample time
delta_f = 1/Ts/FFTSize; % Frequency resolution of FFT 
FreqOffset = OffsetIdx*delta_f/4;% Map offset index back to frequency

== matlab function QAM_16_Transceiver_Nishat/Receiver/Data Decoding/Phase Offset Estimator/Phase Offset Detection ==
  data: In input; Out output
function Out = phasedecision(In)
% Map the estimated phase to one of -pi, -pi/2, 0, pi/2,  
%#codegen
Out = round(In.*2./pi)./2.*pi;
% The above processing is equivalent to the following processing using
% if/else statements
%
% if In<pi/4 && In>-pi/4
%     Out = 0;
% elseif In>=pi/4 && In<pi*3/4
%     Out = pi/2;
% elseif In>=pi*3/4 || In<=-pi*3/4
%     Out = -pi;
% else
%     Out = -pi/2;
% end

== matlab function QAM_16_Transceiver_Nishat/Receiver/Fine Frequency Compensation/PED ==
  data: In input; e output
function e = PED(In)
% Implementation of Maximum Likelihood Phase Error Detector listed in
% Chapter 7.2.2 of "Digital Communications - A Discrete-Time Approach" by
% Michael Rice. This employs a decision directed method.
%
% Input:
%   In - Input samples, oversampled by two
% Output:
%   e - Phase error, de
%#codegen
M=16;
%for 64QAM constillation
if M==64

if real(In)>=0 && real(In)<2
    a=1;
elseif real(In)>=2 && real(In)<4
    a=3;
elseif real(In)>=4 && real(In)<6
    a=5;
elseif real(In)>=6
    a=7;
elseif real(In)<0 && real(In)>-2
    a=-1;
elseif real(In)<=-2 && real(In)>-4
    a=-3;
elseif real(In)<=-4 && real(In)>-6
    a=-5;
else
    a=-7;
end

if imag(In)>=0 && imag(In)<2
    b=1;
elseif imag(In)>=2 && imag(In)<4
    b=3;
elseif imag(In)>=4 && imag(In)<6
    b=5;
elseif imag(In)>=6
    b=7;
elseif imag(In)<0 && imag(In)>-2
    b=-1;
elseif imag(In)<=-2 && imag(In)>-4
    b=-3;
elseif imag(In)<=-4 && imag(In)>-6
    b=-5;
else
    b=-7;
end
r=sqrt(a^2+b^2);

%for 16QAM constillation
elseif M==16

if real(In)>=0 && real(In)<2
    a=1;
elseif real(In)>=2
    a=3;
elseif real(In)<0 && real(In)>=-2
    a=-1;
else
    a=-3;
end

if imag(In)>=0 && imag(In)<2
    b=1;
elseif imag(In)>=2
    b=3;
elseif imag(In)<0 && imag(In)>=-2
    b=-1;
else
    b=-3;

end
r=sqrt(a^2+b^2);

%for 4QAM constillation
else
r=1;

end

  
%R=sqrt(real(In)^2+imag(In)^2);
e =(sign(real(In)).*imag(In) - sign(imag(In)).*real(In))/r;






% function [error,I_hat,Q_hat] = PED(In)
% % Implementation of Maximum Likelihood Phase Error Detector listed in
% % Chapter 7.2.2 of "Digital Communications - A Discrete-Time Approach" by
% % Michael Rice. This employs a decision directed method.
% % 
% % Input: 
% %   In - Input samples, oversampled by two
% % Output:
% %   e - Phase error, de
% %#codegen
% 
% persistent e e1 e2 e3;
% if isempty(e1)
%     e = 0;
%     e1 = 0;
%     e2 = 0;
%     e3 = 0;
% end
% 
% if abs(real(In)) > 2
%     I_hat = sign(real(In))*3;
% else
%     I_hat = sign(real(In))*1;
% end
% 
% if abs(imag(In)) > 2
%     Q_hat = sign(imag(In))*3;
% else
%     Q_hat = sign(imag(In))*1;
% end
% 
% a = sqrt(I_hat^2 + Q_hat^2);
% b = sqrt(real(In)^2 + imag(In)^2);
% 
% if ((a~=0)&&(b~=0))
% e = ( ( I_hat.*imag(In) - Q_hat.*real(In) )/(a*b) );
% else 
%     e = 0;
% end;
% 
% %error = e;
% 
% if ((e> 0.8*e2) &&(e < 1.2*e2))
%     error = e;
% elseif ((e1> 0.8*e3) &&(e1 < 1.2*e3))
%     error = e1;
% else 
%     error = e;
% end
% 
% e3 = e2;
% e2 = e1;
% e1 = e;

== matlab function QAM_16_Transceiver_Nishat/QPSK Receiver/Data Decoding/Phase Offset Estimator/Phase Offset Detection ==
  data: In input; Out output
function Out = phasedecision(In)
% Map the estimated phase to one of -pi, -pi/2, 0, pi/2,  
%#codegen
Out = round(In.*2./pi)./2.*pi;
% The above processing is equivalent to the following processing using
% if/else statements
%
% if In<pi/4 && In>-pi/4
%     Out = 0;
% elseif In>=pi/4 && In<pi*3/4
%     Out = pi/2;
% elseif In>=pi*3/4 || In<=-pi*3/4
%     Out = -pi;
% else
%     Out = -pi/2;
% end

== matlab function QAM_16_Transceiver_Nishat/QPSK Receiver/Fine Frequency Compensation/PED ==
  data: In input; e output
function e = PED(In)
% Implementation of Maximum Likelihood Phase Error Detector listed in
% Chapter 7.2.2 of "Digital Communications - A Discrete-Time Approach" by
% Michael Rice. This employs a decision directed method.
%
% Input:
%   In - Input samples, oversampled by two
% Output:
%   e - Phase error, de
%#codegen
M=16;
%for 64QAM constillation
if M==64

if real(In)>=0 && real(In)<2
    a=1;
elseif real(In)>=2 && real(In)<4
    a=3;
elseif real(In)>=4 && real(In)<6
    a=5;
elseif real(In)>=6
    a=7;
elseif real(In)<0 && real(In)>-2
    a=-1;
elseif real(In)<=-2 && real(In)>-4
    a=-3;
elseif real(In)<=-4 && real(In)>-6
    a=-5;
else
    a=-7;
end

if imag(In)>=0 && imag(In)<2
    b=1;
elseif imag(In)>=2 && imag(In)<4
    b=3;
elseif imag(In)>=4 && imag(In)<6
    b=5;
elseif imag(In)>=6
    b=7;
elseif imag(In)<0 && imag(In)>-2
    b=-1;
elseif imag(In)<=-2 && imag(In)>-4
    b=-3;
elseif imag(In)<=-4 && imag(In)>-6
    b=-5;
else
    b=-7;
end
r=sqrt(a^2+b^2);

%for 16QAM constillation
elseif M==16

if real(In)>=0 && real(In)<2
    a=1;
elseif real(In)>=2
    a=3;
elseif real(In)<0 && real(In)>=-2
    a=-1;
else
    a=-3;
end

if imag(In)>=0 && imag(In)<2
    b=1;
elseif imag(In)>=2
    b=3;
elseif imag(In)<0 && imag(In)>=-2
    b=-1;
else
    b=-3;

end
r=sqrt(a^2+b^2);

%for 4QAM constillation
else
r=1;

end

  
%R=sqrt(real(In)^2+imag(In)^2);
e =(sign(real(In)).*imag(In) - sign(imag(In)).*real(In))/r;






% function [error,I_hat,Q_hat] = PED(In)
% % Implementation of Maximum Likelihood Phase Error Detector listed in
% % Chapter 7.2.2 of "Digital Communications - A Discrete-Time Approach" by
% % Michael Rice. This employs a decision directed method.
% % 
% % Input: 
% %   In - Input samples, oversampled by two
% % Output:
% %   e - Phase error, de
% %#codegen
% 
% persistent e e1 e2 e3;
% if isempty(e1)
%     e = 0;
%     e1 = 0;
%     e2 = 0;
%     e3 = 0;
% end
% 
% if abs(real(In)) > 2
%     I_hat = sign(real(In))*3;
% else
%     I_hat = sign(real(In))*1;
% end
% 
% if abs(imag(In)) > 2
%     Q_hat = sign(imag(In))*3;
% else
%     Q_hat = sign(imag(In))*1;
% end
% 
% a = sqrt(I_hat^2 + Q_hat^2);
% b = sqrt(real(In)^2 + imag(In)^2);
% 
% if ((a~=0)&&(b~=0))
% e = ( ( I_hat.*imag(In) - Q_hat.*real(In) )/(a*b) );
% else 
%     e = 0;
% end;
% 
% %error = e;
% 
% if ((e> 0.8*e2) &&(e < 1.2*e2))
%     error = e;
% elseif ((e1> 0.8*e3) &&(e1 < 1.2*e3))
%     error = e1;
% else 
%     error = e;
% end
% 
% e3 = e2;
% e2 = e1;
% e1 = e;

== matlab function QAM_16_Transceiver_Nishat/Receiver/Timing Recovery/Timing Recovery PLL/Interpolation Filter ==
  data: In input; Out output; mu input
function Out = interp_filter(In, mu)
% Prabolic piecewise polynomial interpolator, Farrow Interpolator with 
% alpha = 1/2, see Figure 8.4.16 of "Digital Communications - A 
% Discrete-Time Approach" by Michael Rice.
% Input:
%   In - Input samples, oversampled by two
%   mu - Difference between actual sampling instant and the optimal instant,
%        between zero and one
% Output:
%   Out - Interpolation output
%#codegen
persistent delay1 delay2 delay3; % Input delayed by 1, 2 and 3 samples
if isempty(delay1)
    [delay1, delay2, delay3] = deal(complex(0,0));
end

K = -0.5;

Out = delay2 + mu.*(K.*(In+delay2+delay3)+(1-K).*delay1)...
      + K.*(delay1+delay2-In-delay3).*mu.^2;
  
% Update delay buffers
delay3 = delay2;
delay2 = delay1;
delay1 = In;

== matlab function QAM_16_Transceiver_Nishat/Receiver/Timing Recovery/Timing Recovery PLL/NCO Control ==
  data: Delta input; Underflow output; mu output; qpsktxrx parameter
function [Underflow, mu] = NCO_ctrl(Delta, qpsktxrx)
% Implementation of modulo-1 counter for interpolation control listed in
% Figure 8.4.19 of "Digital Communications - A Discrete-Time Approach"
% by Michael Rice. See design details in Chapter 8.4.3 of the same book.
% 
% Input:
%   Delta - Loop filter output. If loop is in lock, delta would be small
%   qpsktxrx - Simulation parameter structure
% Output:
%   Underflow - Indicator of counter underflow. This is the strobe signal
%   for downstream processing
%   mu - Difference between actual sampling instant and the optimal instant,
%        between zero and one
%#codegen

% delay1 - Counter value delayed by 1 sample
% Regtemp - The estimated timing error normalized by half QPSK symbols
persistent delay1 Regtemp;  
if isempty(delay1)
    [delay1, Regtemp] = deal(0);
end
Upsampling = qpsktxrx.Upsampling;
Downsampling = qpsktxrx.Downsampling;
oversampling = Upsampling/Downsampling;

counter = mod(delay1,1)-Delta-1/oversampling; % decrementing counter
if counter < 0
    Underflow = 1;
    Regtemp = mod(delay1,1)/(Delta+1/oversampling);
else
    Underflow = 0;
end

mu = Regtemp;

% Update delay buffer
delay1 = mod(delay1,1)-Delta-1/oversampling;

== matlab function QAM_16_Transceiver_Nishat/Receiver/Timing Recovery/Timing Recovery PLL/Timing Error Detector ==
  data: In input; e output; strobe input
function e = TED(In, strobe)
% Zero-Crossing Timing Error Detector. See "Zero-Crossing Timing Error
% Detector" section in Chapter 8.4.1 of "Digital Communications - A
% Discrete-Time Approach" by Michael Rice. For bit stuffing/stripping
% details, see page 490-494 of the same book.
%
% Input: 
%   In - Input samples, interpolation result
%   strobe - Signal to enable timing error calculation
% Output:
%   e - Timing error
%#codegen
persistent delay1 delay2 delayStrobe; % Input delayed by one and 2 samples, and
% Enable signal delayed by one sample
if isempty(delay1)
    [delay1, delay2] = deal(complex(0,0));
    delayStrobe = 0;
end

if strobe==1 && delayStrobe~=strobe
    e = real(delay1) * (sign(real(delay2)) - sign(real(In))) + ...
        imag(delay1) * (sign(imag(delay2)) - sign(imag(In)));
else
    e = 0;
end

if delayStrobe~=strobe
    % Shift contents in delay register
    delay2 = delay1;
    delay1 = In;
elseif strobe==1
    % Two consecutive high strobes
    delay2 = 0; % Stuff missing sample
    delay1 = In; 
end
% If both current and previous enable signals are 0, skip current sample
% and keep the delayed signals unchanged. (Bit stripping)
delayStrobe = strobe;

== matlab function QAM_16_Transceiver_Nishat/QPSK Receiver/Timing Recovery/Calculate Number of Valid Samples ==
  data: Clk input; numValid output
function numValid = numValidCalc(Clk)
% Calculate the number of valid outputs in the current received frame. The
% typical value is 100 valid outputs in a 200-element frame. However, in
% bit stuffing case we have 101 valid outputs, and in bit stripping case we 
% have 99 valid outputs.
%
% Input:
%   Clk - Strobe signal
% Output:
%   NumValid - Number of valid outputs in the current received frame 
%#codegen
numValid = sum(Clk~=0);
